simulink library "Cloudage"  (R2018b)
settings: Solver=ode45  StartTime=0.0  StopTime=10.0  RelTol=1e-3  EnableMultiTasking=on
settings Model: Creator=drhf  LastModifiedBy=P41573
settings DataIOCC: LimitDataPoints=on  SaveFormat=Array  SignalLoggingSaveFormat=ModelDataLogs
settings OptimizationCC: ExpressionDepthLimit=2147483647  LifeSpan=inf
settings DebuggingCC: UnderspecifiedInitializationDetection=Classic  MergeDetectMultiDrivingBlocksExec=none  SolverPrmCheckMsg=warning  FcnCallInpInsideContextMsg=warning  StateNameClashWarn=warning  SFUnexpectedBacktrackingDiag=warning  SFNoUnconditionalDefaultTransitionDiag=warning  SFExecutionAtInitializationDiag=none
settings HardwareCC: ProdBitPerPointer=32  ProdBitPerSizeT=32  ProdBitPerPtrDiffT=32  ProdLargestAtomicFloat=None  ProdIntDivRoundTo=Undefined  ProdEndianess=Unspecified  ProdWordSize=32  ProdHWDeviceType=32-bit Generic
settings ModelReferenceCC: PropagateSignalLabelsOutOfModel=off
settings SFSimCC: SimUseLocalCustomCode=off
settings RTWCC: RTWUseLocalCustomCode=off
settings CodeAppCC: StateflowObjectComments=on
settings GRTTargetCC: TargetLangStandard=C89/C90 (ANSI)  GeneratePreprocessorConditionals=Disable all  CombineOutputUpdateFcns=off  GRTInterface=on
settings ConfigComp: CovMetricSettings=dw  CovHtmlReporting=on  CovSaveCumulativeToWorkspaceVar=on  CovSaveSingleToWorkspaceVar=on  CovExternalEMLEnable=off

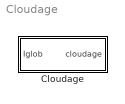
== system Cloudage ==
  Cloudage : Subsystem  mask(cloud index){latitude=51, longitude=-7, longitude0=-30, skytype=high mountain}
      mask prompts: latitude "Latitude [-90;90], north positive"; longitude "Longitude  [-180;180], west positive"; longitude0 "reference longitude (timezone)"; skytype "Sky Type"
      mask help:
      | Calculates the cloud index. The cloud index is the fraction of the sky covered by clouds in [0, 1/8, 2/8, 3/8, ..., 7/8, 1].
      |
      | INPUT VECTOR:
      |  time    : real time or simulation time [s]
      |  Iglob   : global radiation on horizontal surface (W/m²)
      |
      | OUTPUT VECTOR:
      |  cloud  : cloudindex [0;1]
      mask Help: web(fullfile(path_carnot('help'),'Cloudage.html'),'-helpbrowser')
      mask TypeOptions skytype: high mountain | lowland | urban region | industrial zone

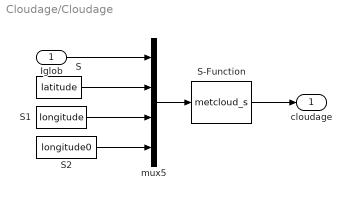
== system Cloudage/Cloudage ==
  Iglob : Inport
  S : Constant  Value=latitude
  S-Function : S-Function  FunctionName=metcloud_s  Parameters=skytype  SFunctionDeploymentMode=off  EnableBusSupport=off
  S1 : Constant  Value=longitude
  S2 : Constant  Value=longitude0
  mux5 : Mux
  cloudage : Outport
  wires:
  Iglob/1 -> mux5/1
  S-Function/1 -> cloudage/1
  S2/1 -> mux5/4
  mux5/1 -> S-Function/1
  S/1 -> mux5/2
  S1/1 -> mux5/3
